simulink model "SprottD_final_2020a"  (R2020a)
settings: Solver=ode23s  StartTime=0.0  StopTime=1000
settings Model: Creator=Ava Hedayatipour  LastModifiedBy=RaviM

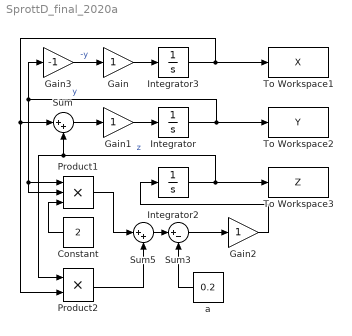
== system SprottD_final_2020a ==
  Constant : Constant  Value=2
  Gain : Gain
  Gain1 : Gain
  Gain2 : Gain
  Gain3 : Gain  Gain=-1
  Integrator : Integrator  InitialCondition=0.7
  Integrator2 : Integrator  InitialCondition=0.4
  Integrator3 : Integrator  InitialCondition=0.1
  Product1 : Product  Inputs=3
  Product2 : Product
  Sum : Sum  Inputs=|++
  Sum3 : Sum  Inputs=|+-
  Sum5 : Sum  Inputs=|++
  To Workspace1 : ToWorkspace  VariableName=X  SaveFormat=Timeseries  SampleTime=-1
  To Workspace2 : ToWorkspace  VariableName=Y  SaveFormat=Timeseries  SampleTime=-1
  To Workspace3 : ToWorkspace  VariableName=Z  SaveFormat=Timeseries  SampleTime=-1
  a : Constant  Value=0.2
  wires:
  Integrator/1 -> Gain3/1, Product1/1, Product1/2, To Workspace2/1  "y"
  Product1/1 -> Sum5/1
  Gain1/1 -> Integrator/1
  Sum5/1 -> Sum3/1
  Gain2/1 -> Integrator2/1
  Integrator3/1 -> To Workspace1/1, Sum/1, Product2/2
  Sum/1 -> Gain1/1
  Sum3/1 -> Gain2/1
  Constant/1 -> Product1/3
  Gain/1 -> Integrator3/1
  Integrator2/1 -> To Workspace3/1, Product2/1, Sum/2  "z"
  Gain3/1 -> Gain/1  "-y"
  a/1 -> Sum3/2
  Product2/1 -> Sum5/2
